simulink model "SeparateAndConcate_img"  (R2016b)
settings: Solver=FixedStepAuto  StartTime=0.0  StopTime=10.0  RelTol=1e-3
libraries: visionsources x1
settings Model: Creator=sk  LastModifiedBy=zeabus
settings SolverCC: PositivePriorityOrder=on
settings OptimizationCC: MaxStackSize=64
settings DebuggingCC: ParameterTunabilityLossMsg=error
settings HardwareCC: ProdBitPerPointer=32  ProdBitPerSizeT=32  ProdBitPerPtrDiffT=32  ProdLargestAtomicInteger=Long  ProdLargestAtomicFloat=Double  ProdWordSize=32  ProdHWDeviceType=ARM Compatible->ARM Cortex
settings RTWCC: SystemTargetFile=ert.tlc  HardwareBoard=Raspberry Pi  TLCOptions="-aInlineSetEventsForThisBaseRateFcn=TLC_FALSE -aSuppressMultiTaskScheduler=TLC_FALSE  -aRateBasedStepFcn=0"  TemplateMakefile=ert_default_tmf  Description=Embedded Coder  GenerateReport=on  Toolchain=GNU GCC Raspberry Pi  IncludeHyperlinkInReport=on  LaunchReport=on  GenerateTraceInfo=on  GenerateTraceReport=on  GenerateTraceReportSl=on  GenerateTraceReportSf=on  GenerateTraceReportEml=on
settings CodeAppCC: ForceParamTrailComments=on  IgnoreCustomStorageClasses=off  OperatorAnnotations=on  SimulinkDataObjDesc=on  SFDataObjDesc=on  MATLABFcnDesc=on  InsertBlockDesc=on  MATLABSourceComments=on
settings ERTTargetCC: SupportVariableSizeSignals=on

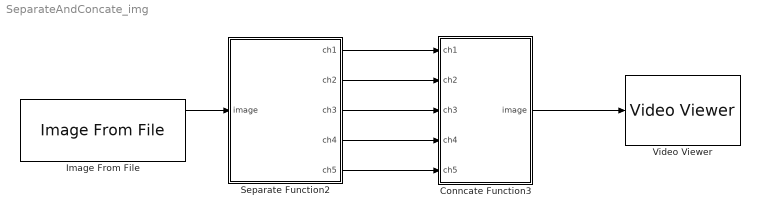
== system SeparateAndConcate_img ==
  Conncate Function3 : MATLAB Function  TreatAsAtomicUnit=on
  Image From File : visionsources/Image From File  Tag=vipblks_nd  FileName=C:\Users\zeabus\Desktop\Workspace\matlab\vision\images\640480.fw.png  imagePorts=Separate color signals  Ts=inf  ImageDataType=Inherit from input image  Signed=on  WordLength=16  sdImageDataType=uint(8)  FractionLengthMode=User-defined  FractionLength=15  OutPortLabels=R|G|B
  Separate Function2 : MATLAB Function  TreatAsAtomicUnit=on
  Video Viewer : VideoViewer  FigPos=[191 761 897 585]
  wires:
  Image From File/1 -> Separate Function2/1(image)
  Conncate Function3/1(image) -> Video Viewer/1
  Separate Function2/1(ch1) -> Conncate Function3/1(ch1)
  Separate Function2/2(ch2) -> Conncate Function3/2(ch2)
  Separate Function2/3(ch3) -> Conncate Function3/3(ch3)
  Separate Function2/4(ch4) -> Conncate Function3/4(ch4)
  Separate Function2/5(ch5) -> Conncate Function3/5(ch5)

== matlab function SeparateAndConcate_img/Conncate Function3 ==
  data: ch1 input; image output; ch2 input; ch3 input; ch4 input; ch5 input
function image = concatenation(ch1,ch2,ch3,ch4,ch5)
maxcol = 128;
ch1 = reshape(ch1,480,maxcol);
ch2 = reshape(ch2,480,maxcol);
ch3 = reshape(ch3,480,maxcol);
ch4 = reshape(ch4,480,maxcol);
ch5 = reshape(ch5,480,maxcol);
image = [ch1,ch2,ch3,ch4,ch5];
image = reshape(image,480,640);

== matlab function SeparateAndConcate_img/Separate Function2 ==
  data: image input; ch1 output; ch2 output; ch3 output; ch4 output; ch5 output
function [ch1,ch2,ch3,ch4,ch5] = separate(image)
maxlength = 61440;
image = reshape(image,1,307200);
ch1 = image(1:maxlength);
ch2 = image(maxlength*1+1:maxlength*2);
ch3 = image(maxlength*2+1:maxlength*3);
ch4 = image(maxlength*3+1:maxlength*4);
ch5 = image(maxlength*4+1:maxlength*5);
